simulink model "gm_FCS_MPC_3Phase_SPMSM_TEST1"  (R2022a)
settings: Solver=ode23t  StartTime=0.0  StopTime=0.2  RelTol=1e-3  AbsTol=1e-3  EnableMultiTasking=on
undefined symbols (not defined in the file or in its folder): f_c, Ld, Lq, np, psiPM, R, T_50MHz, u_dc
libraries: dspsigops x31, hdlmdlgenlib x28, ee_lib x22, nesl_utility x22, fl_lib x21, simulink x7
(part 4 of 5)

== system gm_FCS_MPC_3Phase_SPMSM_TEST1/Microcontroller Software/Subsystem1/MATLAB Function/adder2 ==
  In1 : Inport
  In2 : Inport  Port=2
  adder2 : Sum  OutDataTypeStr=single  SampleTime=1e-10
  adder2_pd1 : Delay  DelayLength=6
  Out1 : Outport
  wires:
  In1/1 -> adder2/1
  In2/1 -> adder2/2
  adder2/1 -> adder2_pd1/1
  adder2_pd1/1 -> Out1/1

== system gm_FCS_MPC_3Phase_SPMSM_TEST1/Microcontroller Software/Subsystem1/MATLAB Function/adder20 ==
  In1 : Inport
  In2 : Inport  Port=2
  adder20 : Sum  OutDataTypeStr=single  SampleTime=1e-10
  adder20_pd1 : Delay  DelayLength=6
  Out1 : Outport
  wires:
  In1/1 -> adder20/1
  In2/1 -> adder20/2
  adder20/1 -> adder20_pd1/1
  adder20_pd1/1 -> Out1/1

== system gm_FCS_MPC_3Phase_SPMSM_TEST1/Microcontroller Software/Subsystem1/MATLAB Function/adder21 ==
  In1 : Inport
  In2 : Inport  Port=2
  adder21 : Sum  OutDataTypeStr=single  SampleTime=1e-10
  adder21_pd1 : Delay  DelayLength=6
  Out1 : Outport
  wires:
  In1/1 -> adder21/1
  In2/1 -> adder21/2
  adder21/1 -> adder21_pd1/1
  adder21_pd1/1 -> Out1/1

== system gm_FCS_MPC_3Phase_SPMSM_TEST1/Microcontroller Software/Subsystem1/MATLAB Function/adder22 ==
  In1 : Inport
  In2 : Inport  Port=2
  adder22 : Sum  OutDataTypeStr=single  SampleTime=1e-10
  adder22_pd1 : Delay  DelayLength=6
  Out1 : Outport
  wires:
  In1/1 -> adder22/1
  In2/1 -> adder22/2
  adder22/1 -> adder22_pd1/1
  adder22_pd1/1 -> Out1/1

== system gm_FCS_MPC_3Phase_SPMSM_TEST1/Microcontroller Software/Subsystem1/MATLAB Function/adder23 ==
  In1 : Inport
  In2 : Inport  Port=2
  adder23 : Sum  OutDataTypeStr=single  SampleTime=1e-10
  adder23_pd1 : Delay  DelayLength=6
  Out1 : Outport
  wires:
  In1/1 -> adder23/1
  In2/1 -> adder23/2
  adder23/1 -> adder23_pd1/1
  adder23_pd1/1 -> Out1/1

== system gm_FCS_MPC_3Phase_SPMSM_TEST1/Microcontroller Software/Subsystem1/MATLAB Function/adder24 ==
  In1 : Inport
  In2 : Inport  Port=2
  adder24 : Sum  OutDataTypeStr=single  SampleTime=1e-10
  adder24_pd1 : Delay  DelayLength=6
  Out1 : Outport
  wires:
  In1/1 -> adder24/1
  In2/1 -> adder24/2
  adder24/1 -> adder24_pd1/1
  adder24_pd1/1 -> Out1/1

== system gm_FCS_MPC_3Phase_SPMSM_TEST1/Microcontroller Software/Subsystem1/MATLAB Function/adder25 ==
  In1 : Inport
  In2 : Inport  Port=2
  adder25 : Sum  OutDataTypeStr=single  SampleTime=1e-10
  adder25_pd1 : Delay  DelayLength=6
  Out1 : Outport
  wires:
  In1/1 -> adder25/1
  In2/1 -> adder25/2
  adder25/1 -> adder25_pd1/1
  adder25_pd1/1 -> Out1/1

== system gm_FCS_MPC_3Phase_SPMSM_TEST1/Microcontroller Software/Subsystem1/MATLAB Function/adder26 ==
  In1 : Inport
  In2 : Inport  Port=2
  adder26 : Sum  OutDataTypeStr=single  SampleTime=1e-10
  adder26_pd1 : Delay  DelayLength=6
  Out1 : Outport
  wires:
  In1/1 -> adder26/1
  In2/1 -> adder26/2
  adder26/1 -> adder26_pd1/1
  adder26_pd1/1 -> Out1/1

== system gm_FCS_MPC_3Phase_SPMSM_TEST1/Microcontroller Software/Subsystem1/MATLAB Function/adder27 ==
  In1 : Inport
  In2 : Inport  Port=2
  adder27 : Sum  OutDataTypeStr=single  SampleTime=1e-10
  adder27_pd1 : Delay  DelayLength=6
  Out1 : Outport
  wires:
  In1/1 -> adder27/1
  In2/1 -> adder27/2
  adder27/1 -> adder27_pd1/1
  adder27_pd1/1 -> Out1/1

== system gm_FCS_MPC_3Phase_SPMSM_TEST1/Microcontroller Software/Subsystem1/MATLAB Function/adder28 ==
  In1 : Inport
  In2 : Inport  Port=2
  adder28 : Sum  OutDataTypeStr=single  SampleTime=1e-10
  adder28_pd1 : Delay  DelayLength=6
  Out1 : Outport
  wires:
  In1/1 -> adder28/1
  In2/1 -> adder28/2
  adder28/1 -> adder28_pd1/1
  adder28_pd1/1 -> Out1/1

== system gm_FCS_MPC_3Phase_SPMSM_TEST1/Microcontroller Software/Subsystem1/MATLAB Function/adder29 ==
  In1 : Inport
  In2 : Inport  Port=2
  adder29 : Sum  OutDataTypeStr=single  SampleTime=1e-10
  adder29_pd1 : Delay  DelayLength=6
  Out1 : Outport
  wires:
  In1/1 -> adder29/1
  In2/1 -> adder29/2
  adder29/1 -> adder29_pd1/1
  adder29_pd1/1 -> Out1/1

== system gm_FCS_MPC_3Phase_SPMSM_TEST1/Microcontroller Software/Subsystem1/MATLAB Function/adder3 ==
  In1 : Inport
  In2 : Inport  Port=2
  adder3 : Sum  OutDataTypeStr=single  SampleTime=1e-10
  adder3_pd1 : Delay  DelayLength=6
  Out1 : Outport
  wires:
  In1/1 -> adder3/1
  In2/1 -> adder3/2
  adder3/1 -> adder3_pd1/1
  adder3_pd1/1 -> Out1/1

== system gm_FCS_MPC_3Phase_SPMSM_TEST1/Microcontroller Software/Subsystem1/MATLAB Function/adder30 ==
  In1 : Inport
  In2 : Inport  Port=2
  adder30 : Sum  OutDataTypeStr=single  SampleTime=1e-10
  adder30_pd1 : Delay  DelayLength=6
  Out1 : Outport
  wires:
  In1/1 -> adder30/1
  In2/1 -> adder30/2
  adder30/1 -> adder30_pd1/1
  adder30_pd1/1 -> Out1/1

== system gm_FCS_MPC_3Phase_SPMSM_TEST1/Microcontroller Software/Subsystem1/MATLAB Function/adder31 ==
  In1 : Inport
  In2 : Inport  Port=2
  adder31 : Sum  OutDataTypeStr=single  SampleTime=1e-10
  adder31_pd1 : Delay  DelayLength=6
  Out1 : Outport
  wires:
  In1/1 -> adder31/1
  In2/1 -> adder31/2
  adder31/1 -> adder31_pd1/1
  adder31_pd1/1 -> Out1/1

== system gm_FCS_MPC_3Phase_SPMSM_TEST1/Microcontroller Software/Subsystem1/MATLAB Function/adder32 ==
  In1 : Inport
  In2 : Inport  Port=2
  adder32 : Sum  OutDataTypeStr=single  SampleTime=1e-10
  adder32_pd1 : Delay  DelayLength=6
  Out1 : Outport
  wires:
  In1/1 -> adder32/1
  In2/1 -> adder32/2
  adder32/1 -> adder32_pd1/1
  adder32_pd1/1 -> Out1/1

== system gm_FCS_MPC_3Phase_SPMSM_TEST1/Microcontroller Software/Subsystem1/MATLAB Function/adder33 ==
  In1 : Inport
  In2 : Inport  Port=2
  adder33 : Sum  OutDataTypeStr=single  SampleTime=1e-10
  adder33_pd1 : Delay  DelayLength=6
  Out1 : Outport
  wires:
  In1/1 -> adder33/1
  In2/1 -> adder33/2
  adder33/1 -> adder33_pd1/1
  adder33_pd1/1 -> Out1/1

== system gm_FCS_MPC_3Phase_SPMSM_TEST1/Microcontroller Software/Subsystem1/MATLAB Function/adder34 ==
  In1 : Inport
  In2 : Inport  Port=2
  adder34 : Sum  OutDataTypeStr=single  SampleTime=1e-10
  adder34_pd1 : Delay  DelayLength=6
  Out1 : Outport
  wires:
  In1/1 -> adder34/1
  In2/1 -> adder34/2
  adder34/1 -> adder34_pd1/1
  adder34_pd1/1 -> Out1/1

== system gm_FCS_MPC_3Phase_SPMSM_TEST1/Microcontroller Software/Subsystem1/MATLAB Function/adder4 ==
  In1 : Inport
  In2 : Inport  Port=2
  adder4 : Sum  OutDataTypeStr=single  SampleTime=1e-10
  adder4_pd1 : Delay  DelayLength=6
  Out1 : Outport
  wires:
  In1/1 -> adder4/1
  In2/1 -> adder4/2
  adder4/1 -> adder4_pd1/1
  adder4_pd1/1 -> Out1/1

== system gm_FCS_MPC_3Phase_SPMSM_TEST1/Microcontroller Software/Subsystem1/MATLAB Function/adder5 ==
  In1 : Inport
  In2 : Inport  Port=2
  adder5 : Sum  OutDataTypeStr=single  SampleTime=1e-10
  adder5_pd1 : Delay  DelayLength=6
  Out1 : Outport
  wires:
  In1/1 -> adder5/1
  In2/1 -> adder5/2
  adder5/1 -> adder5_pd1/1
  adder5_pd1/1 -> Out1/1

== system gm_FCS_MPC_3Phase_SPMSM_TEST1/Microcontroller Software/Subsystem1/MATLAB Function/adder6 ==
  In1 : Inport
  In2 : Inport  Port=2
  adder6 : Sum  OutDataTypeStr=single  SampleTime=1e-10
  adder6_pd1 : Delay  DelayLength=6
  Out1 : Outport
  wires:
  In1/1 -> adder6/1
  In2/1 -> adder6/2
  adder6/1 -> adder6_pd1/1
  adder6_pd1/1 -> Out1/1

== system gm_FCS_MPC_3Phase_SPMSM_TEST1/Microcontroller Software/Subsystem1/MATLAB Function/adder7 ==
  In1 : Inport
  In2 : Inport  Port=2
  adder7 : Sum  OutDataTypeStr=single  SampleTime=1e-10
  adder7_pd1 : Delay  DelayLength=6
  Out1 : Outport
  wires:
  In1/1 -> adder7/1
  In2/1 -> adder7/2
  adder7/1 -> adder7_pd1/1
  adder7_pd1/1 -> Out1/1

== system gm_FCS_MPC_3Phase_SPMSM_TEST1/Microcontroller Software/Subsystem1/MATLAB Function/adder8 ==
  In1 : Inport
  In2 : Inport  Port=2
  adder8 : Sum  OutDataTypeStr=single  SampleTime=1e-10
  adder8_pd1 : Delay  DelayLength=6
  Out1 : Outport
  wires:
  In1/1 -> adder8/1
  In2/1 -> adder8/2
  adder8/1 -> adder8_pd1/1
  adder8_pd1/1 -> Out1/1

== system gm_FCS_MPC_3Phase_SPMSM_TEST1/Microcontroller Software/Subsystem1/MATLAB Function/adder9 ==
  In1 : Inport
  In2 : Inport  Port=2
  adder9 : Sum  OutDataTypeStr=single  SampleTime=1e-10
  adder9_pd1 : Delay  DelayLength=6
  Out1 : Outport
  wires:
  In1/1 -> adder9/1
  In2/1 -> adder9/2
  adder9/1 -> adder9_pd1/1
  adder9_pd1/1 -> Out1/1

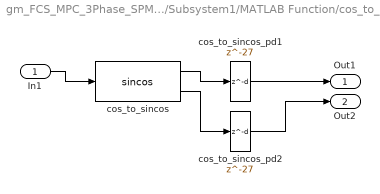
== system gm_FCS_MPC_3Phase_SPMSM_TEST1/Microcontroller Software/Subsystem1/MATLAB Function/cos_to_sincos ==
  In1 : Inport
  cos_to_sincos : Trigonometry  Operator=sincos  SampleTime=1e-10
  cos_to_sincos_pd1 : Delay  DelayLength=27
  cos_to_sincos_pd2 : Delay  DelayLength=27
  Out1 : Outport
  Out2 : Outport  Port=2
  wires:
  In1/1 -> cos_to_sincos/1
  cos_to_sincos/1 -> cos_to_sincos_pd1/1
  cos_to_sincos_pd1/1 -> Out1/1
  cos_to_sincos/2 -> cos_to_sincos_pd2/1
  cos_to_sincos_pd2/1 -> Out2/1

== system gm_FCS_MPC_3Phase_SPMSM_TEST1/Microcontroller Software/Subsystem1/MATLAB Function/gain1 ==
  In1 : Inport
  In2 : Inport  Port=2
  gain1 : Product  Inputs=**  OutDataTypeStr=single  SampleTime=1e-10
  gain1_pd1 : Delay  DelayLength=6
  Out1 : Outport
  wires:
  In1/1 -> gain1/1
  In2/1 -> gain1/2
  gain1/1 -> gain1_pd1/1
  gain1_pd1/1 -> Out1/1

== system gm_FCS_MPC_3Phase_SPMSM_TEST1/Microcontroller Software/Subsystem1/MATLAB Function/multiplier ==
  In1 : Inport
  In2 : Inport  Port=2
  multiplier : Product  Inputs=**  OutDataTypeStr=single  SampleTime=1e-10
  multiplier_pd1 : Delay  DelayLength=6
  Out1 : Outport
  wires:
  In1/1 -> multiplier/1
  In2/1 -> multiplier/2
  multiplier/1 -> multiplier_pd1/1
  multiplier_pd1/1 -> Out1/1

== system gm_FCS_MPC_3Phase_SPMSM_TEST1/Microcontroller Software/Subsystem1/MATLAB Function/multiplier1 ==
  In1 : Inport
  In2 : Inport  Port=2
  multiplier1 : Product  Inputs=**  OutDataTypeStr=single  SampleTime=1e-10
  multiplier1_pd1 : Delay  DelayLength=6
  Out1 : Outport
  wires:
  In1/1 -> multiplier1/1
  In2/1 -> multiplier1/2
  multiplier1/1 -> multiplier1_pd1/1
  multiplier1_pd1/1 -> Out1/1

== system gm_FCS_MPC_3Phase_SPMSM_TEST1/Microcontroller Software/Subsystem1/MATLAB Function/multiplier10 ==
  In1 : Inport
  In2 : Inport  Port=2
  multiplier10 : Product  Inputs=**  OutDataTypeStr=single  SampleTime=1e-10
  multiplier10_pd1 : Delay  DelayLength=6
  Out1 : Outport
  wires:
  In1/1 -> multiplier10/1
  In2/1 -> multiplier10/2
  multiplier10/1 -> multiplier10_pd1/1
  multiplier10_pd1/1 -> Out1/1

== system gm_FCS_MPC_3Phase_SPMSM_TEST1/Microcontroller Software/Subsystem1/MATLAB Function/multiplier100 ==
  In1 : Inport
  In2 : Inport  Port=2
  multiplier100 : Product  Inputs=**  OutDataTypeStr=single  SampleTime=1e-10
  multiplier100_pd1 : Delay  DelayLength=6
  Out1 : Outport
  wires:
  In1/1 -> multiplier100/1
  In2/1 -> multiplier100/2
  multiplier100/1 -> multiplier100_pd1/1
  multiplier100_pd1/1 -> Out1/1

== system gm_FCS_MPC_3Phase_SPMSM_TEST1/Microcontroller Software/Subsystem1/MATLAB Function/multiplier101 ==
  In1 : Inport
  In2 : Inport  Port=2
  multiplier101 : Product  Inputs=**  OutDataTypeStr=single  SampleTime=1e-10
  multiplier101_pd1 : Delay  DelayLength=6
  Out1 : Outport
  wires:
  In1/1 -> multiplier101/1
  In2/1 -> multiplier101/2
  multiplier101/1 -> multiplier101_pd1/1
  multiplier101_pd1/1 -> Out1/1

== system gm_FCS_MPC_3Phase_SPMSM_TEST1/Microcontroller Software/Subsystem1/MATLAB Function/multiplier102 ==
  In1 : Inport
  In2 : Inport  Port=2
  multiplier102 : Product  Inputs=**  OutDataTypeStr=single  SampleTime=1e-10
  multiplier102_pd1 : Delay  DelayLength=6
  Out1 : Outport
  wires:
  In1/1 -> multiplier102/1
  In2/1 -> multiplier102/2
  multiplier102/1 -> multiplier102_pd1/1
  multiplier102_pd1/1 -> Out1/1

== system gm_FCS_MPC_3Phase_SPMSM_TEST1/Microcontroller Software/Subsystem1/MATLAB Function/multiplier103 ==
  In1 : Inport
  In2 : Inport  Port=2
  multiplier103 : Product  Inputs=**  OutDataTypeStr=single  SampleTime=1e-10
  multiplier103_pd1 : Delay  DelayLength=6
  Out1 : Outport
  wires:
  In1/1 -> multiplier103/1
  In2/1 -> multiplier103/2
  multiplier103/1 -> multiplier103_pd1/1
  multiplier103_pd1/1 -> Out1/1

== system gm_FCS_MPC_3Phase_SPMSM_TEST1/Microcontroller Software/Subsystem1/MATLAB Function/multiplier104 ==
  In1 : Inport
  In2 : Inport  Port=2
  multiplier104 : Product  Inputs=**  OutDataTypeStr=single  SampleTime=1e-10
  multiplier104_pd1 : Delay  DelayLength=6
  Out1 : Outport
  wires:
  In1/1 -> multiplier104/1
  In2/1 -> multiplier104/2
  multiplier104/1 -> multiplier104_pd1/1
  multiplier104_pd1/1 -> Out1/1

== system gm_FCS_MPC_3Phase_SPMSM_TEST1/Microcontroller Software/Subsystem1/MATLAB Function/multiplier105 ==
  In1 : Inport
  In2 : Inport  Port=2
  multiplier105 : Product  Inputs=**  OutDataTypeStr=single  SampleTime=1e-10
  multiplier105_pd1 : Delay  DelayLength=6
  Out1 : Outport
  wires:
  In1/1 -> multiplier105/1
  In2/1 -> multiplier105/2
  multiplier105/1 -> multiplier105_pd1/1
  multiplier105_pd1/1 -> Out1/1

== system gm_FCS_MPC_3Phase_SPMSM_TEST1/Microcontroller Software/Subsystem1/MATLAB Function/multiplier106 ==
  In1 : Inport
  In2 : Inport  Port=2
  multiplier106 : Product  Inputs=**  OutDataTypeStr=single  SampleTime=1e-10
  multiplier106_pd1 : Delay  DelayLength=6
  Out1 : Outport
  wires:
  In1/1 -> multiplier106/1
  In2/1 -> multiplier106/2
  multiplier106/1 -> multiplier106_pd1/1
  multiplier106_pd1/1 -> Out1/1

== system gm_FCS_MPC_3Phase_SPMSM_TEST1/Microcontroller Software/Subsystem1/MATLAB Function/multiplier107 ==
  In1 : Inport
  In2 : Inport  Port=2
  multiplier107 : Product  Inputs=**  OutDataTypeStr=single  SampleTime=1e-10
  multiplier107_pd1 : Delay  DelayLength=6
  Out1 : Outport
  wires:
  In1/1 -> multiplier107/1
  In2/1 -> multiplier107/2
  multiplier107/1 -> multiplier107_pd1/1
  multiplier107_pd1/1 -> Out1/1

== system gm_FCS_MPC_3Phase_SPMSM_TEST1/Microcontroller Software/Subsystem1/MATLAB Function/multiplier108 ==
  In1 : Inport
  In2 : Inport  Port=2
  multiplier108 : Product  Inputs=**  OutDataTypeStr=single  SampleTime=1e-10
  multiplier108_pd1 : Delay  DelayLength=6
  Out1 : Outport
  wires:
  In1/1 -> multiplier108/1
  In2/1 -> multiplier108/2
  multiplier108/1 -> multiplier108_pd1/1
  multiplier108_pd1/1 -> Out1/1

== system gm_FCS_MPC_3Phase_SPMSM_TEST1/Microcontroller Software/Subsystem1/MATLAB Function/multiplier109 ==
  In1 : Inport
  In2 : Inport  Port=2
  multiplier109 : Product  Inputs=**  OutDataTypeStr=single  SampleTime=1e-10
  multiplier109_pd1 : Delay  DelayLength=6
  Out1 : Outport
  wires:
  In1/1 -> multiplier109/1
  In2/1 -> multiplier109/2
  multiplier109/1 -> multiplier109_pd1/1
  multiplier109_pd1/1 -> Out1/1

== system gm_FCS_MPC_3Phase_SPMSM_TEST1/Microcontroller Software/Subsystem1/MATLAB Function/multiplier11 ==
  In1 : Inport
  In2 : Inport  Port=2
  multiplier11 : Product  Inputs=**  OutDataTypeStr=single  SampleTime=1e-10
  multiplier11_pd1 : Delay  DelayLength=6
  Out1 : Outport
  wires:
  In1/1 -> multiplier11/1
  In2/1 -> multiplier11/2
  multiplier11/1 -> multiplier11_pd1/1
  multiplier11_pd1/1 -> Out1/1

== system gm_FCS_MPC_3Phase_SPMSM_TEST1/Microcontroller Software/Subsystem1/MATLAB Function/multiplier110 ==
  In1 : Inport
  In2 : Inport  Port=2
  multiplier110 : Product  Inputs=**  OutDataTypeStr=single  SampleTime=1e-10
  multiplier110_pd1 : Delay  DelayLength=6
  Out1 : Outport
  wires:
  In1/1 -> multiplier110/1
  In2/1 -> multiplier110/2
  multiplier110/1 -> multiplier110_pd1/1
  multiplier110_pd1/1 -> Out1/1

== system gm_FCS_MPC_3Phase_SPMSM_TEST1/Microcontroller Software/Subsystem1/MATLAB Function/multiplier111 ==
  In1 : Inport
  In2 : Inport  Port=2
  multiplier111 : Product  Inputs=**  OutDataTypeStr=single  SampleTime=1e-10
  multiplier111_pd1 : Delay  DelayLength=6
  Out1 : Outport
  wires:
  In1/1 -> multiplier111/1
  In2/1 -> multiplier111/2
  multiplier111/1 -> multiplier111_pd1/1
  multiplier111_pd1/1 -> Out1/1

== system gm_FCS_MPC_3Phase_SPMSM_TEST1/Microcontroller Software/Subsystem1/MATLAB Function/multiplier112 ==
  In1 : Inport
  In2 : Inport  Port=2
  multiplier112 : Product  Inputs=**  OutDataTypeStr=single  SampleTime=1e-10
  multiplier112_pd1 : Delay  DelayLength=6
  Out1 : Outport
  wires:
  In1/1 -> multiplier112/1
  In2/1 -> multiplier112/2
  multiplier112/1 -> multiplier112_pd1/1
  multiplier112_pd1/1 -> Out1/1

== system gm_FCS_MPC_3Phase_SPMSM_TEST1/Microcontroller Software/Subsystem1/MATLAB Function/multiplier113 ==
  In1 : Inport
  In2 : Inport  Port=2
  multiplier113 : Product  Inputs=**  OutDataTypeStr=single  SampleTime=1e-10
  multiplier113_pd1 : Delay  DelayLength=6
  Out1 : Outport
  wires:
  In1/1 -> multiplier113/1
  In2/1 -> multiplier113/2
  multiplier113/1 -> multiplier113_pd1/1
  multiplier113_pd1/1 -> Out1/1

== system gm_FCS_MPC_3Phase_SPMSM_TEST1/Microcontroller Software/Subsystem1/MATLAB Function/multiplier114 ==
  In1 : Inport
  In2 : Inport  Port=2
  multiplier114 : Product  Inputs=**  OutDataTypeStr=single  SampleTime=1e-10
  multiplier114_pd1 : Delay  DelayLength=6
  Out1 : Outport
  wires:
  In1/1 -> multiplier114/1
  In2/1 -> multiplier114/2
  multiplier114/1 -> multiplier114_pd1/1
  multiplier114_pd1/1 -> Out1/1

== system gm_FCS_MPC_3Phase_SPMSM_TEST1/Microcontroller Software/Subsystem1/MATLAB Function/multiplier115 ==
  In1 : Inport
  In2 : Inport  Port=2
  multiplier115 : Product  Inputs=**  OutDataTypeStr=single  SampleTime=1e-10
  multiplier115_pd1 : Delay  DelayLength=6
  Out1 : Outport
  wires:
  In1/1 -> multiplier115/1
  In2/1 -> multiplier115/2
  multiplier115/1 -> multiplier115_pd1/1
  multiplier115_pd1/1 -> Out1/1

== system gm_FCS_MPC_3Phase_SPMSM_TEST1/Microcontroller Software/Subsystem1/MATLAB Function/multiplier116 ==
  In1 : Inport
  In2 : Inport  Port=2
  multiplier116 : Product  Inputs=**  OutDataTypeStr=single  SampleTime=1e-10
  multiplier116_pd1 : Delay  DelayLength=6
  Out1 : Outport
  wires:
  In1/1 -> multiplier116/1
  In2/1 -> multiplier116/2
  multiplier116/1 -> multiplier116_pd1/1
  multiplier116_pd1/1 -> Out1/1

== system gm_FCS_MPC_3Phase_SPMSM_TEST1/Microcontroller Software/Subsystem1/MATLAB Function/multiplier117 ==
  In1 : Inport
  In2 : Inport  Port=2
  multiplier117 : Product  Inputs=**  OutDataTypeStr=single  SampleTime=1e-10
  multiplier117_pd1 : Delay  DelayLength=6
  Out1 : Outport
  wires:
  In1/1 -> multiplier117/1
  In2/1 -> multiplier117/2
  multiplier117/1 -> multiplier117_pd1/1
  multiplier117_pd1/1 -> Out1/1

== system gm_FCS_MPC_3Phase_SPMSM_TEST1/Microcontroller Software/Subsystem1/MATLAB Function/multiplier118 ==
  In1 : Inport
  In2 : Inport  Port=2
  multiplier118 : Product  Inputs=**  OutDataTypeStr=single  SampleTime=1e-10
  multiplier118_pd1 : Delay  DelayLength=6
  Out1 : Outport
  wires:
  In1/1 -> multiplier118/1
  In2/1 -> multiplier118/2
  multiplier118/1 -> multiplier118_pd1/1
  multiplier118_pd1/1 -> Out1/1

== system gm_FCS_MPC_3Phase_SPMSM_TEST1/Microcontroller Software/Subsystem1/MATLAB Function/multiplier119 ==
  In1 : Inport
  In2 : Inport  Port=2
  multiplier119 : Product  Inputs=**  OutDataTypeStr=single  SampleTime=1e-10
  multiplier119_pd1 : Delay  DelayLength=6
  Out1 : Outport
  wires:
  In1/1 -> multiplier119/1
  In2/1 -> multiplier119/2
  multiplier119/1 -> multiplier119_pd1/1
  multiplier119_pd1/1 -> Out1/1

== system gm_FCS_MPC_3Phase_SPMSM_TEST1/Microcontroller Software/Subsystem1/MATLAB Function/multiplier12 ==
  In1 : Inport
  In2 : Inport  Port=2
  multiplier12 : Product  Inputs=**  OutDataTypeStr=single  SampleTime=1e-10
  multiplier12_pd1 : Delay  DelayLength=6
  Out1 : Outport
  wires:
  In1/1 -> multiplier12/1
  In2/1 -> multiplier12/2
  multiplier12/1 -> multiplier12_pd1/1
  multiplier12_pd1/1 -> Out1/1

== system gm_FCS_MPC_3Phase_SPMSM_TEST1/Microcontroller Software/Subsystem1/MATLAB Function/multiplier120 ==
  In1 : Inport
  In2 : Inport  Port=2
  multiplier120 : Product  Inputs=**  OutDataTypeStr=single  SampleTime=1e-10
  multiplier120_pd1 : Delay  DelayLength=6
  Out1 : Outport
  wires:
  In1/1 -> multiplier120/1
  In2/1 -> multiplier120/2
  multiplier120/1 -> multiplier120_pd1/1
  multiplier120_pd1/1 -> Out1/1

== system gm_FCS_MPC_3Phase_SPMSM_TEST1/Microcontroller Software/Subsystem1/MATLAB Function/multiplier121 ==
  In1 : Inport
  In2 : Inport  Port=2
  multiplier121 : Product  Inputs=**  OutDataTypeStr=single  SampleTime=1e-10
  multiplier121_pd1 : Delay  DelayLength=6
  Out1 : Outport
  wires:
  In1/1 -> multiplier121/1
  In2/1 -> multiplier121/2
  multiplier121/1 -> multiplier121_pd1/1
  multiplier121_pd1/1 -> Out1/1

== system gm_FCS_MPC_3Phase_SPMSM_TEST1/Microcontroller Software/Subsystem1/MATLAB Function/multiplier122 ==
  In1 : Inport
  In2 : Inport  Port=2
  multiplier122 : Product  Inputs=**  OutDataTypeStr=single  SampleTime=1e-10
  multiplier122_pd1 : Delay  DelayLength=6
  Out1 : Outport
  wires:
  In1/1 -> multiplier122/1
  In2/1 -> multiplier122/2
  multiplier122/1 -> multiplier122_pd1/1
  multiplier122_pd1/1 -> Out1/1

== system gm_FCS_MPC_3Phase_SPMSM_TEST1/Microcontroller Software/Subsystem1/MATLAB Function/multiplier123 ==
  In1 : Inport
  In2 : Inport  Port=2
  multiplier123 : Product  Inputs=**  OutDataTypeStr=single  SampleTime=1e-10
  multiplier123_pd1 : Delay  DelayLength=6
  Out1 : Outport
  wires:
  In1/1 -> multiplier123/1
  In2/1 -> multiplier123/2
  multiplier123/1 -> multiplier123_pd1/1
  multiplier123_pd1/1 -> Out1/1

== system gm_FCS_MPC_3Phase_SPMSM_TEST1/Microcontroller Software/Subsystem1/MATLAB Function/multiplier124 ==
  In1 : Inport
  In2 : Inport  Port=2
  multiplier124 : Product  Inputs=**  OutDataTypeStr=single  SampleTime=1e-10
  multiplier124_pd1 : Delay  DelayLength=6
  Out1 : Outport
  wires:
  In1/1 -> multiplier124/1
  In2/1 -> multiplier124/2
  multiplier124/1 -> multiplier124_pd1/1
  multiplier124_pd1/1 -> Out1/1

== system gm_FCS_MPC_3Phase_SPMSM_TEST1/Microcontroller Software/Subsystem1/MATLAB Function/multiplier125 ==
  In1 : Inport
  In2 : Inport  Port=2
  multiplier125 : Product  Inputs=**  OutDataTypeStr=single  SampleTime=1e-10
  multiplier125_pd1 : Delay  DelayLength=6
  Out1 : Outport
  wires:
  In1/1 -> multiplier125/1
  In2/1 -> multiplier125/2
  multiplier125/1 -> multiplier125_pd1/1
  multiplier125_pd1/1 -> Out1/1

== system gm_FCS_MPC_3Phase_SPMSM_TEST1/Microcontroller Software/Subsystem1/MATLAB Function/multiplier13 ==
  In1 : Inport
  In2 : Inport  Port=2
  multiplier13 : Product  Inputs=**  OutDataTypeStr=single  SampleTime=1e-10
  multiplier13_pd1 : Delay  DelayLength=6
  Out1 : Outport
  wires:
  In1/1 -> multiplier13/1
  In2/1 -> multiplier13/2
  multiplier13/1 -> multiplier13_pd1/1
  multiplier13_pd1/1 -> Out1/1

== system gm_FCS_MPC_3Phase_SPMSM_TEST1/Microcontroller Software/Subsystem1/MATLAB Function/multiplier14 ==
  In1 : Inport
  In2 : Inport  Port=2
  multiplier14 : Product  Inputs=**  OutDataTypeStr=single  SampleTime=1e-10
  multiplier14_pd1 : Delay  DelayLength=6
  Out1 : Outport
  wires:
  In1/1 -> multiplier14/1
  In2/1 -> multiplier14/2
  multiplier14/1 -> multiplier14_pd1/1
  multiplier14_pd1/1 -> Out1/1

== system gm_FCS_MPC_3Phase_SPMSM_TEST1/Microcontroller Software/Subsystem1/MATLAB Function/multiplier15 ==
  In1 : Inport
  In2 : Inport  Port=2
  multiplier15 : Product  Inputs=**  OutDataTypeStr=single  SampleTime=1e-10
  multiplier15_pd1 : Delay  DelayLength=6
  Out1 : Outport
  wires:
  In1/1 -> multiplier15/1
  In2/1 -> multiplier15/2
  multiplier15/1 -> multiplier15_pd1/1
  multiplier15_pd1/1 -> Out1/1

== system gm_FCS_MPC_3Phase_SPMSM_TEST1/Microcontroller Software/Subsystem1/MATLAB Function/multiplier16 ==
  In1 : Inport
  In2 : Inport  Port=2
  multiplier16 : Product  Inputs=**  OutDataTypeStr=single  SampleTime=1e-10
  multiplier16_pd1 : Delay  DelayLength=6
  Out1 : Outport
  wires:
  In1/1 -> multiplier16/1
  In2/1 -> multiplier16/2
  multiplier16/1 -> multiplier16_pd1/1
  multiplier16_pd1/1 -> Out1/1

== system gm_FCS_MPC_3Phase_SPMSM_TEST1/Microcontroller Software/Subsystem1/MATLAB Function/multiplier17 ==
  In1 : Inport
  In2 : Inport  Port=2
  multiplier17 : Product  Inputs=**  OutDataTypeStr=single  SampleTime=1e-10
  multiplier17_pd1 : Delay  DelayLength=6
  Out1 : Outport
  wires:
  In1/1 -> multiplier17/1
  In2/1 -> multiplier17/2
  multiplier17/1 -> multiplier17_pd1/1
  multiplier17_pd1/1 -> Out1/1

== system gm_FCS_MPC_3Phase_SPMSM_TEST1/Microcontroller Software/Subsystem1/MATLAB Function/multiplier18 ==
  In1 : Inport
  In2 : Inport  Port=2
  multiplier18 : Product  Inputs=**  OutDataTypeStr=single  SampleTime=1e-10
  multiplier18_pd1 : Delay  DelayLength=6
  Out1 : Outport
  wires:
  In1/1 -> multiplier18/1
  In2/1 -> multiplier18/2
  multiplier18/1 -> multiplier18_pd1/1
  multiplier18_pd1/1 -> Out1/1

== system gm_FCS_MPC_3Phase_SPMSM_TEST1/Microcontroller Software/Subsystem1/MATLAB Function/multiplier19 ==
  In1 : Inport
  In2 : Inport  Port=2
  multiplier19 : Product  Inputs=**  OutDataTypeStr=single  SampleTime=1e-10
  multiplier19_pd1 : Delay  DelayLength=6
  Out1 : Outport
  wires:
  In1/1 -> multiplier19/1
  In2/1 -> multiplier19/2
  multiplier19/1 -> multiplier19_pd1/1
  multiplier19_pd1/1 -> Out1/1

== system gm_FCS_MPC_3Phase_SPMSM_TEST1/Microcontroller Software/Subsystem1/MATLAB Function/multiplier2 ==
  In1 : Inport
  In2 : Inport  Port=2
  multiplier2 : Product  Inputs=**  OutDataTypeStr=single  SampleTime=1e-10
  multiplier2_pd1 : Delay  DelayLength=6
  Out1 : Outport
  wires:
  In1/1 -> multiplier2/1
  In2/1 -> multiplier2/2
  multiplier2/1 -> multiplier2_pd1/1
  multiplier2_pd1/1 -> Out1/1

== system gm_FCS_MPC_3Phase_SPMSM_TEST1/Microcontroller Software/Subsystem1/MATLAB Function/multiplier20 ==
  In1 : Inport
  In2 : Inport  Port=2
  multiplier20 : Product  Inputs=**  OutDataTypeStr=single  SampleTime=1e-10
  multiplier20_pd1 : Delay  DelayLength=6
  Out1 : Outport
  wires:
  In1/1 -> multiplier20/1
  In2/1 -> multiplier20/2
  multiplier20/1 -> multiplier20_pd1/1
  multiplier20_pd1/1 -> Out1/1

== system gm_FCS_MPC_3Phase_SPMSM_TEST1/Microcontroller Software/Subsystem1/MATLAB Function/multiplier21 ==
  In1 : Inport
  In2 : Inport  Port=2
  multiplier21 : Product  Inputs=**  OutDataTypeStr=single  SampleTime=1e-10
  multiplier21_pd1 : Delay  DelayLength=6
  Out1 : Outport
  wires:
  In1/1 -> multiplier21/1
  In2/1 -> multiplier21/2
  multiplier21/1 -> multiplier21_pd1/1
  multiplier21_pd1/1 -> Out1/1

== system gm_FCS_MPC_3Phase_SPMSM_TEST1/Microcontroller Software/Subsystem1/MATLAB Function/multiplier22 ==
  In1 : Inport
  In2 : Inport  Port=2
  multiplier22 : Product  Inputs=**  OutDataTypeStr=single  SampleTime=1e-10
  multiplier22_pd1 : Delay  DelayLength=6
  Out1 : Outport
  wires:
  In1/1 -> multiplier22/1
  In2/1 -> multiplier22/2
  multiplier22/1 -> multiplier22_pd1/1
  multiplier22_pd1/1 -> Out1/1

== system gm_FCS_MPC_3Phase_SPMSM_TEST1/Microcontroller Software/Subsystem1/MATLAB Function/multiplier23 ==
  In1 : Inport
  In2 : Inport  Port=2
  multiplier23 : Product  Inputs=**  OutDataTypeStr=single  SampleTime=1e-10
  multiplier23_pd1 : Delay  DelayLength=6
  Out1 : Outport
  wires:
  In1/1 -> multiplier23/1
  In2/1 -> multiplier23/2
  multiplier23/1 -> multiplier23_pd1/1
  multiplier23_pd1/1 -> Out1/1

== system gm_FCS_MPC_3Phase_SPMSM_TEST1/Microcontroller Software/Subsystem1/MATLAB Function/multiplier24 ==
  In1 : Inport
  In2 : Inport  Port=2
  multiplier24 : Product  Inputs=**  OutDataTypeStr=single  SampleTime=1e-10
  multiplier24_pd1 : Delay  DelayLength=6
  Out1 : Outport
  wires:
  In1/1 -> multiplier24/1
  In2/1 -> multiplier24/2
  multiplier24/1 -> multiplier24_pd1/1
  multiplier24_pd1/1 -> Out1/1

== system gm_FCS_MPC_3Phase_SPMSM_TEST1/Microcontroller Software/Subsystem1/MATLAB Function/multiplier25 ==
  In1 : Inport
  In2 : Inport  Port=2
  multiplier25 : Product  Inputs=**  OutDataTypeStr=single  SampleTime=1e-10
  multiplier25_pd1 : Delay  DelayLength=6
  Out1 : Outport
  wires:
  In1/1 -> multiplier25/1
  In2/1 -> multiplier25/2
  multiplier25/1 -> multiplier25_pd1/1
  multiplier25_pd1/1 -> Out1/1

== system gm_FCS_MPC_3Phase_SPMSM_TEST1/Microcontroller Software/Subsystem1/MATLAB Function/multiplier26 ==
  In1 : Inport
  In2 : Inport  Port=2
  multiplier26 : Product  Inputs=**  OutDataTypeStr=single  SampleTime=1e-10
  multiplier26_pd1 : Delay  DelayLength=6
  Out1 : Outport
  wires:
  In1/1 -> multiplier26/1
  In2/1 -> multiplier26/2
  multiplier26/1 -> multiplier26_pd1/1
  multiplier26_pd1/1 -> Out1/1

== system gm_FCS_MPC_3Phase_SPMSM_TEST1/Microcontroller Software/Subsystem1/MATLAB Function/multiplier27 ==
  In1 : Inport
  In2 : Inport  Port=2
  multiplier27 : Product  Inputs=**  OutDataTypeStr=single  SampleTime=1e-10
  multiplier27_pd1 : Delay  DelayLength=6
  Out1 : Outport
  wires:
  In1/1 -> multiplier27/1
  In2/1 -> multiplier27/2
  multiplier27/1 -> multiplier27_pd1/1
  multiplier27_pd1/1 -> Out1/1

== system gm_FCS_MPC_3Phase_SPMSM_TEST1/Microcontroller Software/Subsystem1/MATLAB Function/multiplier28 ==
  In1 : Inport
  In2 : Inport  Port=2
  multiplier28 : Product  Inputs=**  OutDataTypeStr=single  SampleTime=1e-10
  multiplier28_pd1 : Delay  DelayLength=6
  Out1 : Outport
  wires:
  In1/1 -> multiplier28/1
  In2/1 -> multiplier28/2
  multiplier28/1 -> multiplier28_pd1/1
  multiplier28_pd1/1 -> Out1/1

== system gm_FCS_MPC_3Phase_SPMSM_TEST1/Microcontroller Software/Subsystem1/MATLAB Function/multiplier29 ==
  In1 : Inport
  In2 : Inport  Port=2
  multiplier29 : Product  Inputs=**  OutDataTypeStr=single  SampleTime=1e-10
  multiplier29_pd1 : Delay  DelayLength=6
  Out1 : Outport
  wires:
  In1/1 -> multiplier29/1
  In2/1 -> multiplier29/2
  multiplier29/1 -> multiplier29_pd1/1
  multiplier29_pd1/1 -> Out1/1

== system gm_FCS_MPC_3Phase_SPMSM_TEST1/Microcontroller Software/Subsystem1/MATLAB Function/multiplier3 ==
  In1 : Inport
  In2 : Inport  Port=2
  multiplier3 : Product  Inputs=**  OutDataTypeStr=single  SampleTime=1e-10
  multiplier3_pd1 : Delay  DelayLength=6
  Out1 : Outport
  wires:
  In1/1 -> multiplier3/1
  In2/1 -> multiplier3/2
  multiplier3/1 -> multiplier3_pd1/1
  multiplier3_pd1/1 -> Out1/1

== system gm_FCS_MPC_3Phase_SPMSM_TEST1/Microcontroller Software/Subsystem1/MATLAB Function/multiplier30 ==
  In1 : Inport
  In2 : Inport  Port=2
  multiplier30 : Product  Inputs=**  OutDataTypeStr=single  SampleTime=1e-10
  multiplier30_pd1 : Delay  DelayLength=6
  Out1 : Outport
  wires:
  In1/1 -> multiplier30/1
  In2/1 -> multiplier30/2
  multiplier30/1 -> multiplier30_pd1/1
  multiplier30_pd1/1 -> Out1/1

== system gm_FCS_MPC_3Phase_SPMSM_TEST1/Microcontroller Software/Subsystem1/MATLAB Function/multiplier31 ==
  In1 : Inport
  In2 : Inport  Port=2
  multiplier31 : Product  Inputs=**  OutDataTypeStr=single  SampleTime=1e-10
  multiplier31_pd1 : Delay  DelayLength=6
  Out1 : Outport
  wires:
  In1/1 -> multiplier31/1
  In2/1 -> multiplier31/2
  multiplier31/1 -> multiplier31_pd1/1
  multiplier31_pd1/1 -> Out1/1

== system gm_FCS_MPC_3Phase_SPMSM_TEST1/Microcontroller Software/Subsystem1/MATLAB Function/multiplier32 ==
  In1 : Inport
  In2 : Inport  Port=2
  multiplier32 : Product  Inputs=**  OutDataTypeStr=single  SampleTime=1e-10
  multiplier32_pd1 : Delay  DelayLength=6
  Out1 : Outport
  wires:
  In1/1 -> multiplier32/1
  In2/1 -> multiplier32/2
  multiplier32/1 -> multiplier32_pd1/1
  multiplier32_pd1/1 -> Out1/1

== system gm_FCS_MPC_3Phase_SPMSM_TEST1/Microcontroller Software/Subsystem1/MATLAB Function/multiplier33 ==
  In1 : Inport
  In2 : Inport  Port=2
  multiplier33 : Product  Inputs=**  OutDataTypeStr=single  SampleTime=1e-10
  multiplier33_pd1 : Delay  DelayLength=6
  Out1 : Outport
  wires:
  In1/1 -> multiplier33/1
  In2/1 -> multiplier33/2
  multiplier33/1 -> multiplier33_pd1/1
  multiplier33_pd1/1 -> Out1/1

== system gm_FCS_MPC_3Phase_SPMSM_TEST1/Microcontroller Software/Subsystem1/MATLAB Function/multiplier34 ==
  In1 : Inport
  In2 : Inport  Port=2
  multiplier34 : Product  Inputs=**  OutDataTypeStr=single  SampleTime=1e-10
  multiplier34_pd1 : Delay  DelayLength=6
  Out1 : Outport
  wires:
  In1/1 -> multiplier34/1
  In2/1 -> multiplier34/2
  multiplier34/1 -> multiplier34_pd1/1
  multiplier34_pd1/1 -> Out1/1

== system gm_FCS_MPC_3Phase_SPMSM_TEST1/Microcontroller Software/Subsystem1/MATLAB Function/multiplier35 ==
  In1 : Inport
  In2 : Inport  Port=2
  multiplier35 : Product  Inputs=**  OutDataTypeStr=single  SampleTime=1e-10
  multiplier35_pd1 : Delay  DelayLength=6
  Out1 : Outport
  wires:
  In1/1 -> multiplier35/1
  In2/1 -> multiplier35/2
  multiplier35/1 -> multiplier35_pd1/1
  multiplier35_pd1/1 -> Out1/1

== system gm_FCS_MPC_3Phase_SPMSM_TEST1/Microcontroller Software/Subsystem1/MATLAB Function/multiplier36 ==
  In1 : Inport
  In2 : Inport  Port=2
  multiplier36 : Product  Inputs=**  OutDataTypeStr=single  SampleTime=1e-10
  multiplier36_pd1 : Delay  DelayLength=6
  Out1 : Outport
  wires:
  In1/1 -> multiplier36/1
  In2/1 -> multiplier36/2
  multiplier36/1 -> multiplier36_pd1/1
  multiplier36_pd1/1 -> Out1/1

== system gm_FCS_MPC_3Phase_SPMSM_TEST1/Microcontroller Software/Subsystem1/MATLAB Function/multiplier37 ==
  In1 : Inport
  In2 : Inport  Port=2
  multiplier37 : Product  Inputs=**  OutDataTypeStr=single  SampleTime=1e-10
  multiplier37_pd1 : Delay  DelayLength=6
  Out1 : Outport
  wires:
  In1/1 -> multiplier37/1
  In2/1 -> multiplier37/2
  multiplier37/1 -> multiplier37_pd1/1
  multiplier37_pd1/1 -> Out1/1

== system gm_FCS_MPC_3Phase_SPMSM_TEST1/Microcontroller Software/Subsystem1/MATLAB Function/multiplier38 ==
  In1 : Inport
  In2 : Inport  Port=2
  multiplier38 : Product  Inputs=**  OutDataTypeStr=single  SampleTime=1e-10
  multiplier38_pd1 : Delay  DelayLength=6
  Out1 : Outport
  wires:
  In1/1 -> multiplier38/1
  In2/1 -> multiplier38/2
  multiplier38/1 -> multiplier38_pd1/1
  multiplier38_pd1/1 -> Out1/1

== system gm_FCS_MPC_3Phase_SPMSM_TEST1/Microcontroller Software/Subsystem1/MATLAB Function/multiplier39 ==
  In1 : Inport
  In2 : Inport  Port=2
  multiplier39 : Product  Inputs=**  OutDataTypeStr=single  SampleTime=1e-10
  multiplier39_pd1 : Delay  DelayLength=6
  Out1 : Outport
  wires:
  In1/1 -> multiplier39/1
  In2/1 -> multiplier39/2
  multiplier39/1 -> multiplier39_pd1/1
  multiplier39_pd1/1 -> Out1/1

== system gm_FCS_MPC_3Phase_SPMSM_TEST1/Microcontroller Software/Subsystem1/MATLAB Function/multiplier4 ==
  In1 : Inport
  In2 : Inport  Port=2
  multiplier4 : Product  Inputs=**  OutDataTypeStr=single  SampleTime=1e-10
  multiplier4_pd1 : Delay  DelayLength=6
  Out1 : Outport
  wires:
  In1/1 -> multiplier4/1
  In2/1 -> multiplier4/2
  multiplier4/1 -> multiplier4_pd1/1
  multiplier4_pd1/1 -> Out1/1

== system gm_FCS_MPC_3Phase_SPMSM_TEST1/Microcontroller Software/Subsystem1/MATLAB Function/multiplier40 ==
  In1 : Inport
  In2 : Inport  Port=2
  multiplier40 : Product  Inputs=**  OutDataTypeStr=single  SampleTime=1e-10
  multiplier40_pd1 : Delay  DelayLength=6
  Out1 : Outport
  wires:
  In1/1 -> multiplier40/1
  In2/1 -> multiplier40/2
  multiplier40/1 -> multiplier40_pd1/1
  multiplier40_pd1/1 -> Out1/1

== system gm_FCS_MPC_3Phase_SPMSM_TEST1/Microcontroller Software/Subsystem1/MATLAB Function/multiplier41 ==
  In1 : Inport
  In2 : Inport  Port=2
  multiplier41 : Product  Inputs=**  OutDataTypeStr=single  SampleTime=1e-10
  multiplier41_pd1 : Delay  DelayLength=6
  Out1 : Outport
  wires:
  In1/1 -> multiplier41/1
  In2/1 -> multiplier41/2
  multiplier41/1 -> multiplier41_pd1/1
  multiplier41_pd1/1 -> Out1/1

== system gm_FCS_MPC_3Phase_SPMSM_TEST1/Microcontroller Software/Subsystem1/MATLAB Function/multiplier42 ==
  In1 : Inport
  In2 : Inport  Port=2
  multiplier42 : Product  Inputs=**  OutDataTypeStr=single  SampleTime=1e-10
  multiplier42_pd1 : Delay  DelayLength=6
  Out1 : Outport
  wires:
  In1/1 -> multiplier42/1
  In2/1 -> multiplier42/2
  multiplier42/1 -> multiplier42_pd1/1
  multiplier42_pd1/1 -> Out1/1

== system gm_FCS_MPC_3Phase_SPMSM_TEST1/Microcontroller Software/Subsystem1/MATLAB Function/multiplier43 ==
  In1 : Inport
  In2 : Inport  Port=2
  multiplier43 : Product  Inputs=**  OutDataTypeStr=single  SampleTime=1e-10
  multiplier43_pd1 : Delay  DelayLength=6
  Out1 : Outport
  wires:
  In1/1 -> multiplier43/1
  In2/1 -> multiplier43/2
  multiplier43/1 -> multiplier43_pd1/1
  multiplier43_pd1/1 -> Out1/1

== system gm_FCS_MPC_3Phase_SPMSM_TEST1/Microcontroller Software/Subsystem1/MATLAB Function/multiplier44 ==
  In1 : Inport
  In2 : Inport  Port=2
  multiplier44 : Product  Inputs=**  OutDataTypeStr=single  SampleTime=1e-10
  multiplier44_pd1 : Delay  DelayLength=6
  Out1 : Outport
  wires:
  In1/1 -> multiplier44/1
  In2/1 -> multiplier44/2
  multiplier44/1 -> multiplier44_pd1/1
  multiplier44_pd1/1 -> Out1/1

== system gm_FCS_MPC_3Phase_SPMSM_TEST1/Microcontroller Software/Subsystem1/MATLAB Function/multiplier45 ==
  In1 : Inport
  In2 : Inport  Port=2
  multiplier45 : Product  Inputs=**  OutDataTypeStr=single  SampleTime=1e-10
  multiplier45_pd1 : Delay  DelayLength=6
  Out1 : Outport
  wires:
  In1/1 -> multiplier45/1
  In2/1 -> multiplier45/2
  multiplier45/1 -> multiplier45_pd1/1
  multiplier45_pd1/1 -> Out1/1

== system gm_FCS_MPC_3Phase_SPMSM_TEST1/Microcontroller Software/Subsystem1/MATLAB Function/multiplier46 ==
  In1 : Inport
  In2 : Inport  Port=2
  multiplier46 : Product  Inputs=**  OutDataTypeStr=single  SampleTime=1e-10
  multiplier46_pd1 : Delay  DelayLength=6
  Out1 : Outport
  wires:
  In1/1 -> multiplier46/1
  In2/1 -> multiplier46/2
  multiplier46/1 -> multiplier46_pd1/1
  multiplier46_pd1/1 -> Out1/1

== system gm_FCS_MPC_3Phase_SPMSM_TEST1/Microcontroller Software/Subsystem1/MATLAB Function/multiplier47 ==
  In1 : Inport
  In2 : Inport  Port=2
  multiplier47 : Product  Inputs=**  OutDataTypeStr=single  SampleTime=1e-10
  multiplier47_pd1 : Delay  DelayLength=6
  Out1 : Outport
  wires:
  In1/1 -> multiplier47/1
  In2/1 -> multiplier47/2
  multiplier47/1 -> multiplier47_pd1/1
  multiplier47_pd1/1 -> Out1/1

== system gm_FCS_MPC_3Phase_SPMSM_TEST1/Microcontroller Software/Subsystem1/MATLAB Function/multiplier48 ==
  In1 : Inport
  In2 : Inport  Port=2
  multiplier48 : Product  Inputs=**  OutDataTypeStr=single  SampleTime=1e-10
  multiplier48_pd1 : Delay  DelayLength=6
  Out1 : Outport
  wires:
  In1/1 -> multiplier48/1
  In2/1 -> multiplier48/2
  multiplier48/1 -> multiplier48_pd1/1
  multiplier48_pd1/1 -> Out1/1

== system gm_FCS_MPC_3Phase_SPMSM_TEST1/Microcontroller Software/Subsystem1/MATLAB Function/multiplier49 ==
  In1 : Inport
  In2 : Inport  Port=2
  multiplier49 : Product  Inputs=**  OutDataTypeStr=single  SampleTime=1e-10
  multiplier49_pd1 : Delay  DelayLength=6
  Out1 : Outport
  wires:
  In1/1 -> multiplier49/1
  In2/1 -> multiplier49/2
  multiplier49/1 -> multiplier49_pd1/1
  multiplier49_pd1/1 -> Out1/1

== system gm_FCS_MPC_3Phase_SPMSM_TEST1/Microcontroller Software/Subsystem1/MATLAB Function/multiplier5 ==
  In1 : Inport
  In2 : Inport  Port=2
  multiplier5 : Product  Inputs=**  OutDataTypeStr=single  SampleTime=1e-10
  multiplier5_pd1 : Delay  DelayLength=6
  Out1 : Outport
  wires:
  In1/1 -> multiplier5/1
  In2/1 -> multiplier5/2
  multiplier5/1 -> multiplier5_pd1/1
  multiplier5_pd1/1 -> Out1/1

== system gm_FCS_MPC_3Phase_SPMSM_TEST1/Microcontroller Software/Subsystem1/MATLAB Function/multiplier50 ==
  In1 : Inport
  In2 : Inport  Port=2
  multiplier50 : Product  Inputs=**  OutDataTypeStr=single  SampleTime=1e-10
  multiplier50_pd1 : Delay  DelayLength=6
  Out1 : Outport
  wires:
  In1/1 -> multiplier50/1
  In2/1 -> multiplier50/2
  multiplier50/1 -> multiplier50_pd1/1
  multiplier50_pd1/1 -> Out1/1

== system gm_FCS_MPC_3Phase_SPMSM_TEST1/Microcontroller Software/Subsystem1/MATLAB Function/multiplier51 ==
  In1 : Inport
  In2 : Inport  Port=2
  multiplier51 : Product  Inputs=**  OutDataTypeStr=single  SampleTime=1e-10
  multiplier51_pd1 : Delay  DelayLength=6
  Out1 : Outport
  wires:
  In1/1 -> multiplier51/1
  In2/1 -> multiplier51/2
  multiplier51/1 -> multiplier51_pd1/1
  multiplier51_pd1/1 -> Out1/1

== system gm_FCS_MPC_3Phase_SPMSM_TEST1/Microcontroller Software/Subsystem1/MATLAB Function/multiplier52 ==
  In1 : Inport
  In2 : Inport  Port=2
  multiplier52 : Product  Inputs=**  OutDataTypeStr=single  SampleTime=1e-10
  multiplier52_pd1 : Delay  DelayLength=6
  Out1 : Outport
  wires:
  In1/1 -> multiplier52/1
  In2/1 -> multiplier52/2
  multiplier52/1 -> multiplier52_pd1/1
  multiplier52_pd1/1 -> Out1/1

== system gm_FCS_MPC_3Phase_SPMSM_TEST1/Microcontroller Software/Subsystem1/MATLAB Function/multiplier53 ==
  In1 : Inport
  In2 : Inport  Port=2
  multiplier53 : Product  Inputs=**  OutDataTypeStr=single  SampleTime=1e-10
  multiplier53_pd1 : Delay  DelayLength=6
  Out1 : Outport
  wires:
  In1/1 -> multiplier53/1
  In2/1 -> multiplier53/2
  multiplier53/1 -> multiplier53_pd1/1
  multiplier53_pd1/1 -> Out1/1

== system gm_FCS_MPC_3Phase_SPMSM_TEST1/Microcontroller Software/Subsystem1/MATLAB Function/multiplier54 ==
  In1 : Inport
  In2 : Inport  Port=2
  multiplier54 : Product  Inputs=**  OutDataTypeStr=single  SampleTime=1e-10
  multiplier54_pd1 : Delay  DelayLength=6
  Out1 : Outport
  wires:
  In1/1 -> multiplier54/1
  In2/1 -> multiplier54/2
  multiplier54/1 -> multiplier54_pd1/1
  multiplier54_pd1/1 -> Out1/1

== system gm_FCS_MPC_3Phase_SPMSM_TEST1/Microcontroller Software/Subsystem1/MATLAB Function/multiplier55 ==
  In1 : Inport
  In2 : Inport  Port=2
  multiplier55 : Product  Inputs=**  OutDataTypeStr=single  SampleTime=1e-10
  multiplier55_pd1 : Delay  DelayLength=6
  Out1 : Outport
  wires:
  In1/1 -> multiplier55/1
  In2/1 -> multiplier55/2
  multiplier55/1 -> multiplier55_pd1/1
  multiplier55_pd1/1 -> Out1/1

== system gm_FCS_MPC_3Phase_SPMSM_TEST1/Microcontroller Software/Subsystem1/MATLAB Function/multiplier56 ==
  In1 : Inport
  In2 : Inport  Port=2
  multiplier56 : Product  Inputs=**  OutDataTypeStr=single  SampleTime=1e-10
  multiplier56_pd1 : Delay  DelayLength=6
  Out1 : Outport
  wires:
  In1/1 -> multiplier56/1
  In2/1 -> multiplier56/2
  multiplier56/1 -> multiplier56_pd1/1
  multiplier56_pd1/1 -> Out1/1

== system gm_FCS_MPC_3Phase_SPMSM_TEST1/Microcontroller Software/Subsystem1/MATLAB Function/multiplier57 ==
  In1 : Inport
  In2 : Inport  Port=2
  multiplier57 : Product  Inputs=**  OutDataTypeStr=single  SampleTime=1e-10
  multiplier57_pd1 : Delay  DelayLength=6
  Out1 : Outport
  wires:
  In1/1 -> multiplier57/1
  In2/1 -> multiplier57/2
  multiplier57/1 -> multiplier57_pd1/1
  multiplier57_pd1/1 -> Out1/1

== system gm_FCS_MPC_3Phase_SPMSM_TEST1/Microcontroller Software/Subsystem1/MATLAB Function/multiplier58 ==
  In1 : Inport
  In2 : Inport  Port=2
  multiplier58 : Product  Inputs=**  OutDataTypeStr=single  SampleTime=1e-10
  multiplier58_pd1 : Delay  DelayLength=6
  Out1 : Outport
  wires:
  In1/1 -> multiplier58/1
  In2/1 -> multiplier58/2
  multiplier58/1 -> multiplier58_pd1/1
  multiplier58_pd1/1 -> Out1/1

== system gm_FCS_MPC_3Phase_SPMSM_TEST1/Microcontroller Software/Subsystem1/MATLAB Function/multiplier59 ==
  In1 : Inport
  In2 : Inport  Port=2
  multiplier59 : Product  Inputs=**  OutDataTypeStr=single  SampleTime=1e-10
  multiplier59_pd1 : Delay  DelayLength=6
  Out1 : Outport
  wires:
  In1/1 -> multiplier59/1
  In2/1 -> multiplier59/2
  multiplier59/1 -> multiplier59_pd1/1
  multiplier59_pd1/1 -> Out1/1

== system gm_FCS_MPC_3Phase_SPMSM_TEST1/Microcontroller Software/Subsystem1/MATLAB Function/multiplier6 ==
  In1 : Inport
  In2 : Inport  Port=2
  multiplier6 : Product  Inputs=**  OutDataTypeStr=single  SampleTime=1e-10
  multiplier6_pd1 : Delay  DelayLength=6
  Out1 : Outport
  wires:
  In1/1 -> multiplier6/1
  In2/1 -> multiplier6/2
  multiplier6/1 -> multiplier6_pd1/1
  multiplier6_pd1/1 -> Out1/1

== system gm_FCS_MPC_3Phase_SPMSM_TEST1/Microcontroller Software/Subsystem1/MATLAB Function/multiplier60 ==
  In1 : Inport
  In2 : Inport  Port=2
  multiplier60 : Product  Inputs=**  OutDataTypeStr=single  SampleTime=1e-10
  multiplier60_pd1 : Delay  DelayLength=6
  Out1 : Outport
  wires:
  In1/1 -> multiplier60/1
  In2/1 -> multiplier60/2
  multiplier60/1 -> multiplier60_pd1/1
  multiplier60_pd1/1 -> Out1/1

== system gm_FCS_MPC_3Phase_SPMSM_TEST1/Microcontroller Software/Subsystem1/MATLAB Function/multiplier61 ==
  In1 : Inport
  In2 : Inport  Port=2
  multiplier61 : Product  Inputs=**  OutDataTypeStr=single  SampleTime=1e-10
  multiplier61_pd1 : Delay  DelayLength=6
  Out1 : Outport
  wires:
  In1/1 -> multiplier61/1
  In2/1 -> multiplier61/2
  multiplier61/1 -> multiplier61_pd1/1
  multiplier61_pd1/1 -> Out1/1

== system gm_FCS_MPC_3Phase_SPMSM_TEST1/Microcontroller Software/Subsystem1/MATLAB Function/multiplier62 ==
  In1 : Inport
  In2 : Inport  Port=2
  multiplier62 : Product  Inputs=**  OutDataTypeStr=single  SampleTime=1e-10
  multiplier62_pd1 : Delay  DelayLength=6
  Out1 : Outport
  wires:
  In1/1 -> multiplier62/1
  In2/1 -> multiplier62/2
  multiplier62/1 -> multiplier62_pd1/1
  multiplier62_pd1/1 -> Out1/1

== system gm_FCS_MPC_3Phase_SPMSM_TEST1/Microcontroller Software/Subsystem1/MATLAB Function/multiplier63 ==
  In1 : Inport
  In2 : Inport  Port=2
  multiplier63 : Product  Inputs=**  OutDataTypeStr=single  SampleTime=1e-10
  multiplier63_pd1 : Delay  DelayLength=6
  Out1 : Outport
  wires:
  In1/1 -> multiplier63/1
  In2/1 -> multiplier63/2
  multiplier63/1 -> multiplier63_pd1/1
  multiplier63_pd1/1 -> Out1/1

== system gm_FCS_MPC_3Phase_SPMSM_TEST1/Microcontroller Software/Subsystem1/MATLAB Function/multiplier64 ==
  In1 : Inport
  In2 : Inport  Port=2
  multiplier64 : Product  Inputs=**  OutDataTypeStr=single  SampleTime=1e-10
  multiplier64_pd1 : Delay  DelayLength=6
  Out1 : Outport
  wires:
  In1/1 -> multiplier64/1
  In2/1 -> multiplier64/2
  multiplier64/1 -> multiplier64_pd1/1
  multiplier64_pd1/1 -> Out1/1

== system gm_FCS_MPC_3Phase_SPMSM_TEST1/Microcontroller Software/Subsystem1/MATLAB Function/multiplier65 ==
  In1 : Inport
  In2 : Inport  Port=2
  multiplier65 : Product  Inputs=**  OutDataTypeStr=single  SampleTime=1e-10
  multiplier65_pd1 : Delay  DelayLength=6
  Out1 : Outport
  wires:
  In1/1 -> multiplier65/1
  In2/1 -> multiplier65/2
  multiplier65/1 -> multiplier65_pd1/1
  multiplier65_pd1/1 -> Out1/1

== system gm_FCS_MPC_3Phase_SPMSM_TEST1/Microcontroller Software/Subsystem1/MATLAB Function/multiplier66 ==
  In1 : Inport
  In2 : Inport  Port=2
  multiplier66 : Product  Inputs=**  OutDataTypeStr=single  SampleTime=1e-10
  multiplier66_pd1 : Delay  DelayLength=6
  Out1 : Outport
  wires:
  In1/1 -> multiplier66/1
  In2/1 -> multiplier66/2
  multiplier66/1 -> multiplier66_pd1/1
  multiplier66_pd1/1 -> Out1/1

== system gm_FCS_MPC_3Phase_SPMSM_TEST1/Microcontroller Software/Subsystem1/MATLAB Function/multiplier67 ==
  In1 : Inport
  In2 : Inport  Port=2
  multiplier67 : Product  Inputs=**  OutDataTypeStr=single  SampleTime=1e-10
  multiplier67_pd1 : Delay  DelayLength=6
  Out1 : Outport
  wires:
  In1/1 -> multiplier67/1
  In2/1 -> multiplier67/2
  multiplier67/1 -> multiplier67_pd1/1
  multiplier67_pd1/1 -> Out1/1

== system gm_FCS_MPC_3Phase_SPMSM_TEST1/Microcontroller Software/Subsystem1/MATLAB Function/multiplier68 ==
  In1 : Inport
  In2 : Inport  Port=2
  multiplier68 : Product  Inputs=**  OutDataTypeStr=single  SampleTime=1e-10
  multiplier68_pd1 : Delay  DelayLength=6
  Out1 : Outport
  wires:
  In1/1 -> multiplier68/1
  In2/1 -> multiplier68/2
  multiplier68/1 -> multiplier68_pd1/1
  multiplier68_pd1/1 -> Out1/1

== system gm_FCS_MPC_3Phase_SPMSM_TEST1/Microcontroller Software/Subsystem1/MATLAB Function/multiplier69 ==
  In1 : Inport
  In2 : Inport  Port=2
  multiplier69 : Product  Inputs=**  OutDataTypeStr=single  SampleTime=1e-10
  multiplier69_pd1 : Delay  DelayLength=6
  Out1 : Outport
  wires:
  In1/1 -> multiplier69/1
  In2/1 -> multiplier69/2
  multiplier69/1 -> multiplier69_pd1/1
  multiplier69_pd1/1 -> Out1/1

== system gm_FCS_MPC_3Phase_SPMSM_TEST1/Microcontroller Software/Subsystem1/MATLAB Function/multiplier7 ==
  In1 : Inport
  In2 : Inport  Port=2
  multiplier7 : Product  Inputs=**  OutDataTypeStr=single  SampleTime=1e-10
  multiplier7_pd1 : Delay  DelayLength=6
  Out1 : Outport
  wires:
  In1/1 -> multiplier7/1
  In2/1 -> multiplier7/2
  multiplier7/1 -> multiplier7_pd1/1
  multiplier7_pd1/1 -> Out1/1

== system gm_FCS_MPC_3Phase_SPMSM_TEST1/Microcontroller Software/Subsystem1/MATLAB Function/multiplier70 ==
  In1 : Inport
  In2 : Inport  Port=2
  multiplier70 : Product  Inputs=**  OutDataTypeStr=single  SampleTime=1e-10
  multiplier70_pd1 : Delay  DelayLength=6
  Out1 : Outport
  wires:
  In1/1 -> multiplier70/1
  In2/1 -> multiplier70/2
  multiplier70/1 -> multiplier70_pd1/1
  multiplier70_pd1/1 -> Out1/1

== system gm_FCS_MPC_3Phase_SPMSM_TEST1/Microcontroller Software/Subsystem1/MATLAB Function/multiplier71 ==
  In1 : Inport
  In2 : Inport  Port=2
  multiplier71 : Product  Inputs=**  OutDataTypeStr=single  SampleTime=1e-10
  multiplier71_pd1 : Delay  DelayLength=6
  Out1 : Outport
  wires:
  In1/1 -> multiplier71/1
  In2/1 -> multiplier71/2
  multiplier71/1 -> multiplier71_pd1/1
  multiplier71_pd1/1 -> Out1/1

== system gm_FCS_MPC_3Phase_SPMSM_TEST1/Microcontroller Software/Subsystem1/MATLAB Function/multiplier72 ==
  In1 : Inport
  In2 : Inport  Port=2
  multiplier72 : Product  Inputs=**  OutDataTypeStr=single  SampleTime=1e-10
  multiplier72_pd1 : Delay  DelayLength=6
  Out1 : Outport
  wires:
  In1/1 -> multiplier72/1
  In2/1 -> multiplier72/2
  multiplier72/1 -> multiplier72_pd1/1
  multiplier72_pd1/1 -> Out1/1
